simulink model "PrimeraEcuacionSimulink"  (R2023b)
settings: Solver=VariableStepAuto  StartTime=0.0  StopTime=60  RelTol=1e-3
settings Model: LastModifiedBy=Nico Narvaez

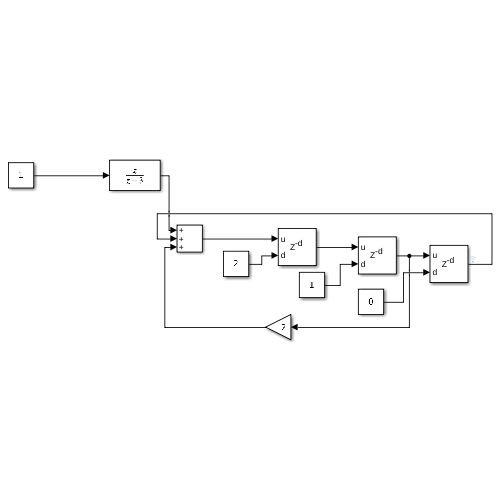
[thumbnail: Simulink's stored preview of the top-level diagram]
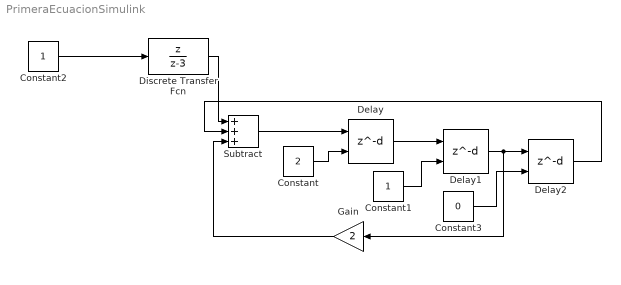
== system PrimeraEcuacionSimulink ==
  Constant : Constant  Value=2
  Constant1 : Constant
  Constant2 : Constant
  Constant3 : Constant  Value=0
  Delay : Delay  DelayLengthSource=Input port  DelayLength=1  InitialCondition=0
      settings: InputPortMap=u0,p1
  Delay1 : Delay  DelayLengthSource=Input port  DelayLength=1  InitialCondition=0
      settings: InputPortMap=u0,p1
  Delay2 : Delay  DelayLengthSource=Input port  DelayLength=1  InitialCondition=0
      settings: InputPortMap=u0,p1
  Discrete Transfer Fcn : DiscreteTransferFcn  Numerator=[1 0]  Denominator=[1 -3]
  Gain : Gain  Gain=2
  Subtract : Sum  Inputs=+++
  wires:
  Delay2/1 -> Subtract/2
  Discrete Transfer Fcn/1 -> Subtract/1
  Delay1/1 -> Gain/1, Delay2/1
  Constant3/1 -> Delay2/2
  Delay/1 -> Delay1/1
  Gain/1 -> Subtract/3
  Constant2/1 -> Discrete Transfer Fcn/1
  Constant1/1 -> Delay1/2
  Subtract/1 -> Delay/1
  Constant/1 -> Delay/2
